simulink model "curiosity_i2c_pitch_roll_yaw"  (R2025b)
settings: Solver=FixedStepDiscrete  StartTime=0.0  StopTime=inf  FixedStep=1e-3  RelTol=1e-3  EnableMultiTasking=on
undefined symbols (not defined in the file): A0, ADC, D10, D7, D8, D9, DiscIntNeverNeededParam, Max, MaxPer, ms, NumBits1, NumBits2, P1, P58, P59, Pin, Resol, s, Timer, us
libraries: MCHP_Blockset x18, simulink x17
(part 1 of 4)
settings Model: SimulationMode=external  ExtModeEnableFloating=off  ExtModeTrigDuration=20  Creator=I52209  LastModifiedBy=I67977
settings SolverCC: AlgebraicLoopSolver=TrustRegion
settings OptimizationCC: DefaultParameterBehavior=Inlined  DefaultUnderspecifiedDataType=single  EnhancedBackFolding=on  BooleansAsBitfields=on  PassReuseOutputArgsAs=Individual arguments  ZeroExternalMemoryAtStartup=off  ZeroInternalMemoryAtStartup=off  OptimizeBlockOrder=speed  DifferentSizesBufferReuse=on  EfficientTunableParamExpr=on
settings DebuggingCC: MultiTaskDSMMsg=none  MultiTaskCondExecSysMsg=none  MultiTaskRateTransMsg=warning  ParameterTunabilityLossMsg=error  ArithmeticOperatorsInVariantConditions=warning
settings HardwareCC: ProdBitPerPointer=32.0  ProdBitPerSizeT=32.0  ProdBitPerPtrDiffT=32.0  ProdLargestAtomicInteger=Long  ProdWordSize=32.0  ProdLongLongMode=on  ProdHWDeviceType=Generic->Custom
settings ModelReferenceCC: ModelReferenceNumInstancesAllowed=Single
settings SFSimCC: MATLABDynamicMemAlloc=off  CustomCodeUndefinedFunction=UseInterfaceOnly
settings RTWCC: SystemTargetFile=MCHP_dsPIC33A_noTMF_stf.tlc  TLCOptions="-aExtModeXCPClassicInterface=0  -aCreateExtModeTypes=1 -aExtModeXCPSimulationTimeInTicks=1"  TemplateMakefile=MCHP_dsPIC33A.tmf  Toolchain=MPLAB XC-DSC - v3.21 for dsPIC DSCs (Microchip)  BuildConfiguration=Specify  GPUComputeCapability=3.5  Description=Microchip Embedded Target dsPIC33A no TMF (real-time)
settings CodeAppCC: ForceParamTrailComments=on  IgnoreCustomStorageClasses=off  MaxIdLength=255.0  OperatorAnnotations=on  SimulinkDataObjDesc=on  SFDataObjDesc=on  InsertBlockDesc=on
settings STFCustomTargetCC: SystemTargetFile=MCHP_dsPIC33A_noTMF_stf.tlc  TargetLangStandard=C99 (ISO)  MultiwordLength=256.0  ConcurrentExecutionCompliant=off  CombineOutputUpdateFcns=on  CombineSignalStateStructs=on  ERTCustomFileBanners=on  SupportContinuousTime=off  RemoveResetFunc=on  MATLABClassNameForMDSCustomization=Simulink.SoftwareTarget.ERTCustomization  GRTInterface=off  UseToolchainInfoCompliant=on  TIMER_PERIOD="[0  49999  65535]"  LDFLAGS='--report-mem,-Map=$(PRODUCT_NAME).map,-cref,-lq-dsp,--memorysummary,memoryfile.xml'  TIMER_START="[0  3  0]"  MCHP_MULTITHREAD_COMPILATION=on  OPTIM_GCC=-O2 -fno-short-double -mno-eds-warn -mconst-in-data -mlarge-code -mlarge-data -mlarge-aggregate -g -Wa,--reorder  OBJDUMP=xc-dsc-objdump  RTWGenSettings_txt="s.UART_TX_IMPLEMENTATION='[2]';s.UART_RX_IMPLEMENTATION='[2]';s.UART_TX_DMACHANNEL='[0]';s.UART_HALF_DUPLEX_MODE='[0]';s.UART_TX_THREAD_PROTECTION='[9]';s.RefMasterBlk='curiosity_i2c_pitch_roll_yaw/CuriosityPlatform Development Board dsPIC33AK128MC106 GP DIM/Microchip Master';s.ChipIdN='[33  128  106]';s.ChipIdL1='AK';s.ChipIdL2='MC';s.ChipIdL3=' ';s.arch3='33A';s.ChipId='33AK128MC106';s.Arch='8';s.bitFieldsSFR='3';s.ChipRAM='16384';s.ChipRAM_XBegin='16384';s.ChipRAM_dma='[-1 -1]';s.FuseConfigTxt='#pragma config FWDT_WDTEN = SW\\\\n#pragma config FICD_JTAGEN = OFF\\\\n#pragma config FDEVOPT_ALTI2C2 = ON\\\\n';s.TimeStep_Timer='2';s.TimeStep_SyncADC='1';s.ADPCFG='0';s.ANSEL_Exist='1';s.ANSEL='[4031   975    -1    -1    -1    -1    -1    -1    -1    -1    -1]';s.TRIS='[65535  65535  63495  65535     -1     -1     -1     -1     -1     -1     -1     -1     -1     -1     -1     -1     -1     -1     -1     -1     -1     -1     -1     -1     -1     -1     -1     -1     -1     -1     -1     -1     -1     -1     -1     -1     -1     -1     -1     -1     -1     -1     -1     -1     -1     -1     -1     -1     -1     -1     -1     -1     -1     -1     -1     -1     -1]';s.RPOR='[-1    -1    -1    -1    -1    -1    -1    -1    -1    -1    -1    -1    -1    -1  2304    -1    -1    -1    -1    -1]';s.RPINR='[-1  -1  -1  -1  -1  -1  -1  -1  -1  59  -1  -1  -1  -1  -1  -1  -1  -1  -1  -1  -1  -1]';s.LATSET='[-1 -1 -1 -1 -1 -1 -1 -1 -1 -1 -1 -1 -1 -1 -1 -1 -1 -1 -1 -1 -1 -1 -1 -1 -1 -1 -1 -1 -1 -1 -1 -1 -1 -1 -1 -1 -1 -1 -1 -1 -1 -1 -1 -1 -1 -1 -1 -1 -1 -1 -1 -1 -1 -1 -1 -1 -1]';s.LATCLR='[-1 -1 -1 -1 -1 -1 -1 -1 -1 -1 -1 -1 -1 -1 -1 -1 -1 -1 -1 -1 -1 -1 -1 -1 -1 -1 -1 -1 -1 -1 -1 -1 -1 -1 -1 -1 -1 -1 -1 -1 -1 -1 -1 -1 -1 -1 -1 -1 -1 -1 -1 -1 -1 -1 -1 -1 -1]';s.ODC='[-1 -1 -1 -1 -1 -1 -1 -1 -1 -1 -1 -1 -1 -1 -1 -1 -1 -1 -1 -1 -1 -1 -1 -1 -1 -1 -1 -1 -1 -1 -1 -1 -1 -1 -1 -1 -1 -1 -1 -1 -1 -1 -1 -1 -1 -1 -1 -1 -1 -1 -1 -1 -1 -1 -1 -1 -1]';s.CNPU='[-1 -1 -1 -1 -1 -1 -1 -1 -1 -1 -1 -1 -1 -1 -1 -1 -1 -1 -1 -1 -1 -1 -1 -1 -1 -1 -1 -1 -1 -1 -1 -1 -1 -1 -1 -1 -1 -1 -1 -1 -1 -1 -1 -1 -1 -1 -1 -1 -1 -1 -1 -1 -1 -1 -1 -1 -1]';s.CNPD='[-1 -1 -1 -1 -1 -1 -1 -1 -1 -1 -1 -1 -1 -1 -1 -1 -1 -1 -1 -1 -1 -1 -1 -1 -1 -1 -1 -1 -1 -1 -1 -1 -1 -1 -1 -1 -1 -1 -1 -1 -1 -1 -1 -1 -1 -1 -1 -1 -1 -1 -1 -1 -1 -1 -1 -1 -1]';s.PortConfigTxt=' ';s.CLKDIV='0';s.PLLFBD='-1';s.PLLDIV='16815713';s.QUARTZ='8000000';s.SWITCH_OSC='16386';s.PLLRNG='-1';s.MASTER_BusyFlag='-1';s.POWERSAVE='0';s.MIPS='200000000';s.FLASH_ECC='0';s.PBxDIV='[-1]';s.CLKx_INTDIV='[-1 -1 -1 -1  0  1 -1  0  0 -1 -1  0 -1]';s.CLKx_FRACDIV='[-1   -1   -1   -1    0  256   -1    0    0   -1   -1    0   -1]';s.AN_type2='1';s.ACLKCON_reg='-1';s.nTIMERS='1';s.nSCCP='4';s.DOS_04094_cpu_33a_v1_dspic33a='1';s.DOS_04436_perseus_dspic33a='1';s.DOS_04928_gpio_ports_upb_v2_dspic33a='1';s.DOS_02672_math_progcrc_upb_v1_dspic33a='1';s.DOS_04993_sec_32bit_cp_upb_v1_dspic33a='1';s.DOS_03459_adc_pc_ctrl_upb_v2_dspic33a='1';s.DOS_04302_pwm_pc_upb_v3_dspic33a='1';s.DOS_03076_uart_protocol_upb_v1_dspic33a='1';s.DOS_01482_spi_i2s_upb_v1_dspic33a='1';s.DOS_05155_i2c_upb_v4_dspic33a='1';s.DOS_02359_sent_j2716_upb_v1_dspic33a='1';s.DOS_05177_qei_32b_upb_v2_dspic33a='1';s.DOS_01512_ccp_mccp_upb_v1_dspic33a='1';s.DOS_03496_dac_pdm_nbit_upb_v2_dspic33a='1';s.DOS_02673_tmr_classa_upb_v1_dspic33a='1';s.DOS_04776_perf_mon_upb_v1_dspic33a='1';s.DOS_03680_pfm_pbu_33a_upb_v1_dspic33a='1';s.DOS_04649_sec_pac_upb_v0_dspic33a='1';s.DOS_03966_io_integrity_monitor_upb_v1_dspic33a='1';s.DOS_04641_biss_master_upb_v1_dspic33a='1';s.DOS_04077_dma_upb_v1_dspic33a='1';s.DOS_04549_nvm_ctrl_32bit_upb_v1_dspic33a='1';s.DOS_04449_clk_cru_33a_upb_v1_dspic33a='1';s.DOS_03850_clk_monitor_upb_v1_dspic33a='1';s.DOS_04342_osc_rc8mhz_ctrl_upb_v4_dspic33a='1';s.DOS_04650_wdt_upb_v4_dspic33a='1';s.DOS_05178_ptg_pc_upb_v2_dspic33a='1';s.DOS_04181_data_ram_ctrl_upb_v1_dspic33a='1';s.DOS_04735_wdt_dmt_upb_v6_dspic33a='1';s.DOS_01577_cla_clc_upb_v1_dspic33a='1';s.DOS_03516_pwr_sib_upb_v3_dspic33a='1';s.DOS_03495_amp_pad_opamp_ctrl_upb_v2_dspic33a='1';s.DOS_05308_pegasus_dspic33a='0';s.DOS_02976_adc_12b_upb_v2_dspic33a='0';s.DOS_05404_adc_pc_ctrl_upb_v3_dspic33a='0';s.DOS_05226_pwm_pc_upb_v4_dspic33a='0';s.DOS_05226_apwm_pc_upb_v4_dspic33a='0';s.DOS_05431_dac_pdm_nbit_upb_v3_dspic33a='0';s.DOS_04649_sec_pac_upb_v1_dspic33a='0';s.DOS_05461_pwr_sib_upb_v4_dspic33a='0';s.DOS_05420_amp_vref_ctl_upb_v1_dspic33a='0';s.DOS_05346_sec_cam_v2_dspic33a='0';s.DOS_03267_adc_soft_code_seq_v1_dspic33a='0';s.DOS_04537_can_fd_upb_v3_dspic33a='0';s.DOS_05557_serpens_dspic33a='0';s.DOS_05972_adc_12b_upb_v3_adc_dspic33a='0';s.DOS_03681_bmx_33a_upb_v1_dspic33a='0';s.DOS_05514_qei_32b_upb_v3_dspic33a='0';s.DOS_02050_tmr_rtcc_upb_v1_dspic33a='0';s.DOS_04649_sec_pac_upb_serpens_dspic33a='0';s.DOS_05801_dma_upb_v2_dspic33a='0';s.DOS_05692_pwr_sib_upb_v5_dspic33a='0';s.DOS_06006_adc_soft_code_seq_v2_adc_dspic33a='0';s.DOS_05442_icd_trace_33a_v1_dspic33a='0';s.DOS_02551_cpu_16bit_v7='0';s.DOS_01520_wdt_dmt_upb_v1_16bit='0';s.DOS_02359a_sent_j2716_upb_v1='0';s.DOS_02672_math_progcrc_upb_v1_16bit='0';s.DOS_01577_cla_clc_upb_v1='0';s.DOS_02915_ecc_v2='0';s.DOS_02673_tmr_classa_upb_v1_16bit='0';s.DOS_01494_qei_32b_upb_v1_16bit='0';s.DOS_02472_ppi_pmp16_upb_v1_16bit='0';s.DOS_01441_i2c_upb_v1_16bit_TLAH='0';s.DOS_03076_uart_protocol_upb_v1_16bit='0';s.DOS_01482='0';s.DOS_01483_pwm_16bit='0';s.DOS_02949_WACG='0';s.DOS_02316_nvm_ctrl_v1_16bit='0';s.DOS_03349_amp_pad_opamp_ctrl_upb_v1='0';s.DOS_02653_afe_current_bias_ctrl_upb_v1_16bit='0';s.DOS_01459_ptg_pc_upb_v1_16bit='0';s.DOS_01512_ccp_mccp_upb_v1_16bit='0';s.DOS_02519_dma_sfr_16bit_v2='0';s.DOS_02508c11='0';s.DOS_02475_dac_pdm_nbit_upb_v1_16bit='0';s.DOS_02467_gpio_upb_v1_16bit='0';s.DOS_00805_rst_integration_v4='0';s.DOS_02659_clk_sib_v12='0';s.DOS_02237_osc_dco_ctrl_upb_v1_16bit='0';s.DOS_02674_wdt_upb_v1_16bit='0';s.DOS_01407='0';s.DOS_03247_CAN_FD_UPB_V2_16_bit='0';s.DOS_03994_WAC07='0';s.DOS_02552_msi_upb_v1_Master='0';s.DOS_03667_pwm_pc_upb_v2_16bit='0';s.DOS_04180_drm_ctrl_ecc_v1='0';s.DOS_03431_STX03='0';s.DOS_03516_pwr_sib_upb_v3='0';s.DOS_02552_msi_upb_v1_Slave='0';s.DOS_04621_amp_pga_ctrl_upb_v3='0';s.DOS_02497_WACV='0';s.DOS_02593_amp_pga_ctrl_pb_v2_16bit='0';s.DOS_01461_afe_ctmu_con_upb_v1_16bit='0';s.DOS_02497_WACA='0';s.DOS_02478_uart_irda_upb_v1_16bit='0';s.DOS_00929='0';s.DOS_01198='0';s.DOS_03029_WACH='0';s.DOS_01483_apwm_16bit='0';s.DOS_04797_WAC0A='0';s.DOS_04884_WAC0B='0';s.DOS_04797_WAC09='0';s.DOS_03662_WACU='0';s.DOS_00794='0';s.DOS_00931='0';s.DOS_00932='0';s.DOS_00942='0';s.DOS_00938='0';s.DOS_00996='0';s.DOS_00997='0';s.DOS_00998='0';s.DOS_00209='0';s.DOS_01555_adc='0';s.DOS_01293='0';s.DOS_00828='0';s.DOS_01116='0';s.DOS_01017_RPORx='0';s.DOS_01017_RPINRx='0';s.DOS_01555_nvm_tsmc18_v2_16bit='0';s.DOS_00804='0';s.DOS_00826='0';s.DOS_01555_TLAK_PMDx='0';s.DOS_01555_TLAK_INT_='0';s.DOS_00933='0';s.DOS_01555='0';s.DOS_01555_ptg='0';s.DOS_00958='0';s.DOS_01117_PORTx='0';s.DOS_00999='0';s.DOS_01041='0';s.DOS_00892='0';s.DOS_01287_TLAC_PMDx='0';s.DOS_01287_TLAC_INT_='0';s.DOS_01424='0';s.DOS_01332='0';s.DOS_01468_PMBA_current_source='0';s.DOS_02291_PGA='0';s.DOS_01467_Comparator='0';s.DOS_01498_TLAY='0';s.DOS_00993_PLL_120MHz='0';s.DOS_01332_ptg_pc_v1='0';s.DOS_00958_pwm_TLAY='0';s.TLAY_IOPorts='0';s.DOS_00929q='0';s.DOS_02415_spi_v5='0';s.DOS_RPINRx_16bit_2='0';s.DOS_01497_TLAH_PMDx='0';s.DOS_02550_TLAL_INT='0';s.DOS_00958_pwm_TLAH='0';s.DOS_01287_TLAH_INT_='0';s.DOS_01113='0';s.DOS_01017_PMDx='0';s.DOS_00927='0';s.DOS_01080='0';s.DOS_00794_cpu_16bit_v3='0';s.DOS_02192_TLCD_PMDx='0';s.DOS_02192_TLCD_INT_='0';s.DOS_02192_cmp='0';s.DOS_00958_pwm_TLCD='0';s.DOS_02192_PORTx_TLCD='0';s.DOS_00936='0';s.DOS_00995='0';s.DOS_00546='0';s.DOS_00474='0';s.DOS_02481_WACP_Config='0';s.DOS_03088_pfm_cache_ocp_v2_WACK='0';s.DOS_02819_pfm_ctrl_32bit_upb_v2='0';s.DOS_02674_wdt_upb_v1_32bit='0';s.DOS_01520_wdt_dmt_upb_v1='0';s.DOS_02869_icd_jtag_bvci_upb_v2='0';s.DOS_02823_WACJ_clk_cru_upb_v2='0';s.DOS_02823_WACN_clk_cru_upb_v2='0';s.DOS_01423_RPINRx='0';s.DOS_02481_RPORx='0';s.DOS_02511_pwr_sib_upb_v1_32bit='0';s.DOS_02907_WACP_int_evic_v3='0';s.DOS_01500_dma_bvci_v2='0';s.DOS_02141_tmr_classa_pb_v2='0';s.DOS_02815_tmr_classb_upb_v1='0';s.DOS_00740_icap_pb_v1='0';s.DOS_00749_ocmp_pb_v1='0';s.DOS_01441_i2c_upb_v1_32bit='0';s.DOS_01329_spi_pb_v2='0';s.DOS_02478_uart_irda_upb_v1_32bit='0';s.DOS_01477_pwm_mc_upb_v1='0';s.DOS_01494_qei_32b_upb_v1='0';s.DOS_03554_cmp_control_upb_v2_32bit='0';s.DOS_01445_dac_nbit__control_upb_v1_32bit='0';s.DOS_01461_afe_ctmu_con_upb_v1='0';s.DOS_01577_cla_clc_upb_v1_32bit='0';s.DOS_02467_gpio_ports_upb_v1='0';s.DOS_02508_WACP_adc_sar_ctrl_upb_v1='0';s.DOS_01261_tmr_rtcc_WACJ_K_N_P_pb_v2='0';s.DOS_EIP_00136_ssx_v1='0';s.DOS_02481_WACK_MC_Config='0';s.DOS_02907_WACN_GP_int_evic_v3='0';s.DOS_02508_adc_sar_ctrl_upb_v1_PIC32MK='0';s.DOS_01261_tmr_rtcc_pb_v2='0';s.DOS_01475_lpwr_deep_sleep_ctrl_v2='0';s.DOS_02907_WACN_MC_int_evic_v3='0';s.DOS_03247_can_fd_upb_v2_pic32mk='0';s.DOS_02907_WACK_MC_int_evic_v3='0';s.DOS_02514_dfm_strl_sst_upb_v1='0';s.DOS_02472_ppi_pmp16_upb_v1='0';s.DOS_02813a_usb_otgcore_pb_v3='0';s.DOS_02481_WACJ_MC_Config='0';s.DOS_02569_pfm_cache_ocp_v1='0';s.DOS_02481_WACJ_MC_int_evic_v3='0';s.DOS_01459_ptg_pc_upb_v1_SIC='0';s.DOS_01427_cmp_control_upb_v1_32bit='0';s.DOS_01152_can_bvci_v1='0';s.DOS_02787_WACD_Config='0';s.DOS_00800_dac_4bit_ctrl_pb_v1='0';s.DOS_01539_icd_jtag_pb_v2='0';s.DOS_02823_clk_cru_upb_v2='0';s.DOS_01423_RPORx='0';s.DOS_02907_WACD_int_evic_v3='0';s.DOS_00734_uart_irda_pb_v1='0';s.DOS_00687_tmr_classa_pb_v1='0';s.DOS_00745_tmr_classb_pb_v1='0';s.DOS_02508_adc_sar_ctrl_upb_v1='0';s.DOS_00866_cmp_control_pb_v2='0';s.DOS_01114_eth_bvci_v1='0';s.DOS_02831_usb_clk_rst_v2='0';s.DOS_01643_pfm_cache_ahb_v2='0';s.DOS_EIP_00206r5_sqi_v2='0';s.DOS_EIP_00124_usb_hs_otgcore_v1='0';s.DOS_EIP_00218_math_rng_ahbs_v2='0';s.DOS_EIP_00109_ebi_v1='0';s.DOS_EIP_00158_crypto_v1='0';"  PIC_REF=33AK128MC106  BIN2HEX=xc-dsc-bin2hex  AR1=xc-dsc-ar  GCCPATH=C:/PROGRA~1/MICROC~1/xc-dsc/v3.21/bin  MCHP_AUTO_FLASH=off  LINKER_SCRIPT=p33AK128MC106.gld  MCHP_XCP_MemoryBlockParameters=[-1 8]  AssemblyListing=on  LinkWithMaster=off  TIMER_PRESCALER="[-1  1  1 -1 -1]"  ProduceHexOutput=off  EXTMODE_DATA_UPLOAD=on  HOST_PLATFORM=PC  GCC1=xc-dsc-gcc.exe
settings ERTTargetCC: ExtMode=on  ExtModeTransport=1.0  ExtModeStaticAlloc=on  ExtModeMaxTrigDuration=20.0  ExtModeStaticAllocSize=2048.0  ExtModeMexFile=ext_xcp  ExtModeMexArgs=1 21 460800 './curiosity_i2c_pitch_roll_yaw.X/curiosity_i2c_pitch_roll_yaw.elf'  ExtModeIntrfLevel=Level2 - Open  ERTSrcFileBannerTemplate=MCHP_dsPIC_code_template.cgt  ERTHdrFileBannerTemplate=MCHP_dsPIC_code_template.cgt  ERTDataSrcFileTemplate=MCHP_dsPIC_code_template.cgt  ERTDataHdrFileTemplate=MCHP_dsPIC_code_template.cgt  ERTCustomFileTemplate=MCHP_main.tlc  MaxLineWidth=110.0  TargetLangStandard=C99 (ISO)  ParMdlRefBuildCompliant=off  CompOptLevelCompliant=off  ConcurrentExecutionCompliant=off  CombineSignalStateStructs=on  SupportNonInlinedSFcns=on  ModelStepFunctionPrototypeControlCompliant=off  CPPClassGenCompliant=off

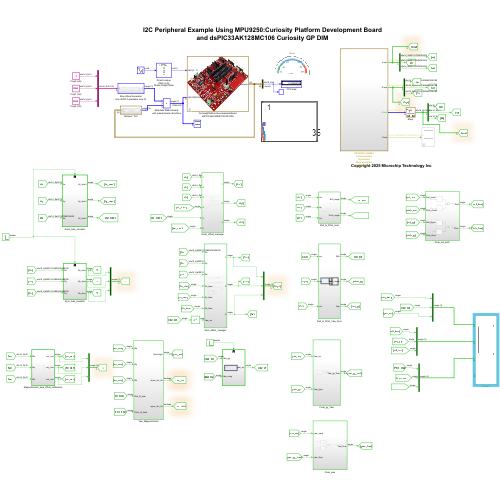
[thumbnail: Simulink's stored preview of the top-level diagram]
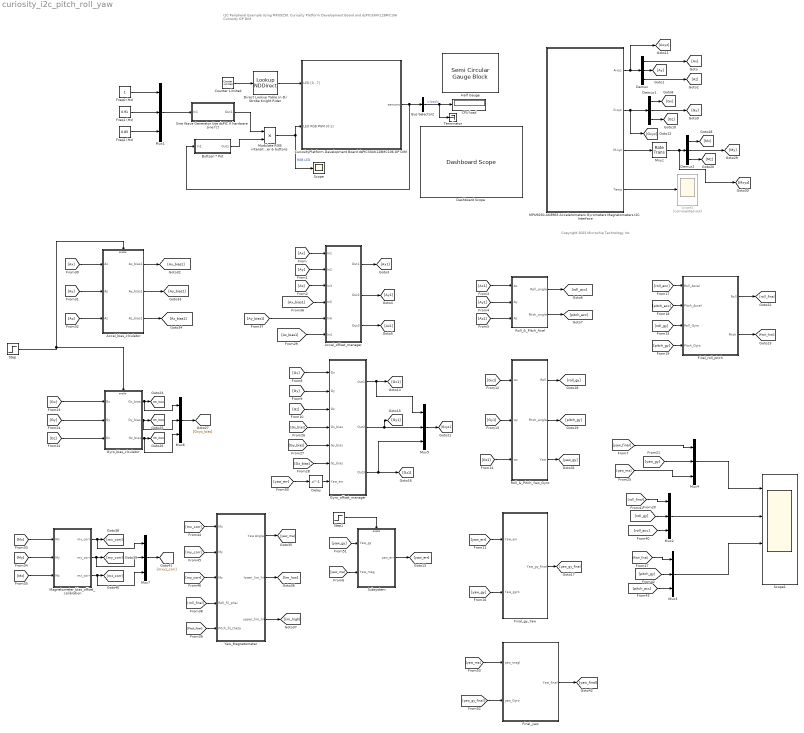
== system curiosity_i2c_pitch_roll_yaw ==
  note: Copyright 2025 Microchip Technology Inc
  note: I2C Peripheral Example Using MPU9250: Curiosity Platform Development Board and dsPIC33AK128MC106 Curiosity GP DIM
  Accel_bias_clculator : Subsystem  TreatAsAtomicUnit=on
  Accel_offset_manager : Subsystem
  Bus Selector2 : BusSelector  OutputSignals=MCU.load
  Buttosn * Pot : Subsystem
  CPU load : Display
  Counter Limited : simulink/Sources/Counter Limited  uplimit=13  tsamp=0.05
  CuriosityPlatform Development Board dsPIC33AK128MC106 GP DIM : Subsystem
      mask Display: image('MCHP_i_Board_Curiosity_dsPICA.jpg')
  Dashboard Scope : DashboardScope  TimeSpan=5  Ymin=0  Ymax=1  LegendPosition=Hide  ScaleAtStop=off  TicksPosition=Inside  FontColor=[0.0, 0.0, 0.0]
  Delay : Delay  DelayLength=1
  Demux : Demux  Outputs=3
  Demux1 : Demux  Outputs=3
  Demux2 : Demux  Outputs=3
  Direct Lookup Table (n-D) Strobe Knight Rider : LookupNDDirect  NumberOfTableDimensions=1  Table=uint16(2.^[[0:7] [6:-1:1]] )  RemoveProtectionInput=on
  Final_gy_Yaw : Subsystem
  Final_roll_pitch : Subsystem
  Final_yaw : Subsystem
  Freq0 (Hz) : Constant  OutDataTypeStr=fixdt(0,16,10)
  Freq1 (Hz) : Constant  Value=0.91  OutDataTypeStr=fixdt(0,16,10)
  Freq2 (Hz) : Constant  Value=0.85  OutDataTypeStr=fixdt(0,16,10)
  Gyro_bias_clculator : Subsystem  TreatAsAtomicUnit=on
  Gyro_offset_manager : Subsystem
  Half Gauge : SemiCircularGaugeBlock  FontColor=[0.0, 0.0, 0.0]
  MPU9250-AK8963 Accelerometers Gyrometers Magnetometers I2C Interface : Subsystem
  Magnetometer_bias_offset_calibration : Subsystem  TreatAsAtomicUnit=on
  Modulate RGB intensity with potentiometer & buttons : Product  OutDataTypeStr=single
  Mux{1..7} (7 alike) : Mux  Inputs=3
  Mxyz : RateTransition  Deterministic=off  OutPortSampleTimeOpt=Inherit
  Roll_&_Pitch_Acel : Subsystem
  Roll_&_Pitch_Yaw_Gyro : Subsystem
  Scope : Scope
      settings: ActiveDisplayYMinimum=-0.06269  ActiveDisplayYMaximum=0.5642
  Scope1 : Scope  NumInputPorts=4
      settings: ActiveDisplayYMinimum=-0.37342479638755322  ActiveDisplayYMaximum=0.911760849878192  DataLoggingVariableName=ScopeData2
  Scope2 : Scope  Commented=on
      settings: ActiveDisplayYMinimum=19.60574  ActiveDisplayYMaximum=33.5483  DataLoggingVariableName=ScopeData3
  Sine Wave Generator Use dsPIC A hardware sine fct : Subsystem
  Step : Step  Time=2  Before=1  After=0  SampleTime=0.005
  Step1 : Step  Time=2  Before=1  After=0  SampleTime=0.005
  Subsystem : Subsystem
  Terminator : Terminator
  Yaw_Magnetometer : Subsystem
  wires:
  [Gy] -> Gyro_offset_manager/2(Gy)
  [yaw_gy] -> Mux4/2
  [Ay] -> Accel_offset_manager/2(In2)
  [Gz] -> Gyro_offset_manager/3(Gz)
  MPU9250-AK8963 Accelerometers Gyrometers Magnetometers I2C Interface/2(G-xyz) -> [Gxyz], Demux1/1
  [Gy] -> Gyro_bias_clculator/2(Gy)
  Yaw_Magnetometer/3(upper_lim_hit) -> [lim_high]
  [Az1] -> Roll_&_Pitch_Acel/3(Az)
  Demux1/2 -> [Gy]
  Mux6/1 -> [Gxyz_bias]
  [yaw_ma] -> Final_yaw/1(yaw_magl)
  [yaw_gy] -> Subsystem/1(Yaw_gy)
  [pitch_gy] -> Final_roll_pitch/4(Pitch_Gyro)
  Magnetometer_bias_offset_calibration/3(mz_corr) -> Mux7/3, [mz_corr]
  [roll_final] -> Mux2/1
  Counter Limited/1 -> Direct Lookup Table (n-D) Strobe Knight Rider/1
  [Ay_bias1] -> Accel_offset_manager/5(In6)
  [yaw_ma] -> Mux4/3
  [Gz] -> Gyro_bias_clculator/3(Gz)
  [Gx_bias] -> Gyro_offset_manager/4(Gx_bias)
  [mz_corr] -> Yaw_Magnetometer/3(Mz)
  Yaw_Magnetometer/1(Yaw Angle) -> [yaw_ma]
  Accel_bias_clculator/2(Ay_bias1) -> [Ay_bias1]
  Demux2/1 -> [Mx]
  [mx_corr] -> Yaw_Magnetometer/1(Mx)
  [yaw_gy_final] -> Final_yaw/2(yaw_Gyro)
  Demux2/2 -> [My]
  [yaw_ma] -> Subsystem/2(Yaw_mag)
  Sine Wave Generator Use dsPIC A hardware sine fct/1(Out1) -> Modulate RGB intensity with potentiometer & buttons/1
  Final_yaw/1(Yaw_final) -> [yaw_final]
  Demux1/1 -> [Gx]
  Gyro_bias_clculator/1(Gx_bias) -> Mux6/1, [Gx_bias]
  [roll_gy] -> Mux2/2
  [Ax] -> Accel_offset_manager/1(In1)
  Buttosn * Pot/1(Out1) -> Modulate RGB intensity with potentiometer & buttons/2
  Modulate RGB intensity with potentiometer & buttons/1 -> CuriosityPlatform Development Board dsPIC33AK128MC106 GP DIM/2(LED RGB PWM [0-1]), Scope/1  "RGB LED"
  Roll_&_Pitch_Yaw_Gyro/3(Yaw) -> [yaw_gy]
  [roll_acc] -> Mux2/3
  Freq2 (Hz)/1 -> Mux1/3
  Final_gy_Yaw/1(Yaw_gy_final) -> [yaw_gy_final]
  Freq0 (Hz)/1 -> Mux1/1
  Step/1 -> Accel_bias_clculator/Enable, Gyro_bias_clculator/Enable
  [Az] -> Accel_offset_manager/3(In3)
  [pitch_acc] -> Final_roll_pitch/2(Pitch_Accel)
  Magnetometer_bias_offset_calibration/2(my_corr) -> Mux7/2, [my_corr]
  [Gz_bias] -> Gyro_offset_manager/6(Gz_bias)
  [pitch_acc] -> Mux3/3
  Yaw_Magnetometer/2(lower_lim_hit) -> [lim_low]
  Demux2/3 -> [Mz]
  Gyro_offset_manager/2(Out2) -> [Gy1], Mux5/2
  [My] -> Magnetometer_bias_offset_calibration/2(My)
  Step1/1 -> Subsystem/Enable
  Demux/2 -> [Ay]
  Gyro_offset_manager/1(Out1) -> [Gx1], Mux5/1
  [yaw_err] -> Final_gy_Yaw/1(Yaw_err)
  Mxyz/1 -> [Mxyz], Demux2/1
  CuriosityPlatform Development Board dsPIC33AK128MC106 GP DIM/1(sensors) -> Buttosn * Pot/1(In1), Bus Selector2/1
  [Gy_bias] -> Gyro_offset_manager/5(Gy_bias)
  [roll_gy] -> Final_roll_pitch/3(Roll_Gyro)
  Accel_bias_clculator/1(Ax_bias1) -> [Ax_bias1]
  [Mz] -> Magnetometer_bias_offset_calibration/3(Mz)
  [Az] -> Accel_bias_clculator/3(Az)
  Roll_&_Pitch_Acel/1(Roll_angle) -> [roll_acc]
  [Az_bias1] -> Accel_offset_manager/6(In4)
  Mux4/1 -> Scope1/1
  [roll_final] -> Yaw_Magnetometer/4(Roll_fil_phai)
  Bus Selector2/1 -> Terminator/1, CPU load/1  "<load>"
  [my_corr] -> Yaw_Magnetometer/2(My)
  [yaw_final] -> Mux4/1
  [Gy1] -> Roll_&_Pitch_Yaw_Gyro/2(wy)
  Demux1/3 -> [Gz]
  [Gx] -> Gyro_bias_clculator/1(Gx)
  [Ax_bias1] -> Accel_offset_manager/4(In5)
  Roll_&_Pitch_Yaw_Gyro/2(Pitch_angle) -> [pitch_gy]
  Gyro_bias_clculator/3(Gz_bias) -> Mux6/3, [Gz_bias]
  Mux3/1 -> Scope1/3
  [Pitch_final] -> Yaw_Magnetometer/5(Pitch_fil_theta)
  Magnetometer_bias_offset_calibration/1(mx_corr) -> Mux7/1, [mx_corr]
  Accel_offset_manager/1(Out1) -> [Ax1]
  [Ax1] -> Roll_&_Pitch_Acel/1(Ax)
  [Mx] -> Magnetometer_bias_offset_calibration/1(Mx)
  Accel_offset_manager/3(Out3) -> [Az1]
  [Ax] -> Accel_bias_clculator/1(Ax)
  [yaw_err] -> Delay/1
  Demux/3 -> [Az]
  Subsystem/1(yaw_err) -> [yaw_err]
  Mux1/1 -> Sine Wave Generator Use dsPIC A hardware sine fct/1(In1)
  [Gx] -> Gyro_offset_manager/1(Gx)
  Roll_&_Pitch_Yaw_Gyro/1(Roll) -> [roll_gy]
  MPU9250-AK8963 Accelerometers Gyrometers Magnetometers I2C Interface/3(M-xyz) -> Mxyz/1
  Gyro_bias_clculator/2(Gy_bias) -> Mux6/2, [Gy_bias]
  Mux2/1 -> Scope1/2
  MPU9250-AK8963 Accelerometers Gyrometers Magnetometers I2C Interface/1(A-xyz) -> Demux/1, [Axyz]
  [yaw_gy] -> Final_gy_Yaw/2(Yaw_gyro)
  [Ay] -> Accel_bias_clculator/2(Ay)
  [Gz1] -> Roll_&_Pitch_Yaw_Gyro/3(wz)
  Demux/1 -> [Ax]
  [Gx1] -> Roll_&_Pitch_Yaw_Gyro/1(wx)
  [Pitch_final] -> Mux3/1
  MPU9250-AK8963 Accelerometers Gyrometers Magnetometers I2C Interface/4(Temp) -> Scope2/1
  Direct Lookup Table (n-D) Strobe Knight Rider/1 -> CuriosityPlatform Development Board dsPIC33AK128MC106 GP DIM/1(LED [0...7])
  Delay/1 -> Gyro_offset_manager/7(Yaw_err)
  Final_roll_pitch/2(Pitch) -> [Pitch_final]
  Accel_bias_clculator/3(Az_bias1) -> [Az_bias1]
  Final_roll_pitch/1(Roll) -> [roll_final]
  Freq1 (Hz)/1 -> Mux1/2
  Accel_offset_manager/2(Out2) -> [Ay1]
  [pitch_gy] -> Mux3/2
  Roll_&_Pitch_Acel/2(Pitch_angle) -> [pitch_acc]
  Gyro_offset_manager/3(Out3) -> Mux5/3, [Gz1]
  Mux5/1 -> [Gxyz1]
  [roll_acc] -> Final_roll_pitch/1(Roll_Accel)
  Mux7/1 -> [mxyz_corr]
  [Ay1] -> Roll_&_Pitch_Acel/2(Ay)

== system curiosity_i2c_pitch_roll_yaw/Accel_bias_clculator ==
  Ax : Inport
  Ay : Inport  Port=2
  Az : Inport  Port=3
  Enable : EnablePort
  manu_mean : Subsystem
  manu_mean3 : Subsystem
  manu_mean4 : Subsystem
  Ax_bias1 : Outport
  Ay_bias1 : Outport  Port=2
  Az_bias1 : Outport  Port=3
  wires:
  Ay/1 -> manu_mean3/1(Ay)
  Ax/1 -> manu_mean/1(Ax)
  Az/1 -> manu_mean4/1(Az)
  manu_mean/1(Ax_bias1) -> Ax_bias1/1
  manu_mean3/1(Ay_bias1) -> Ay_bias1/1
  manu_mean4/1(Ax_bias1) -> Az_bias1/1

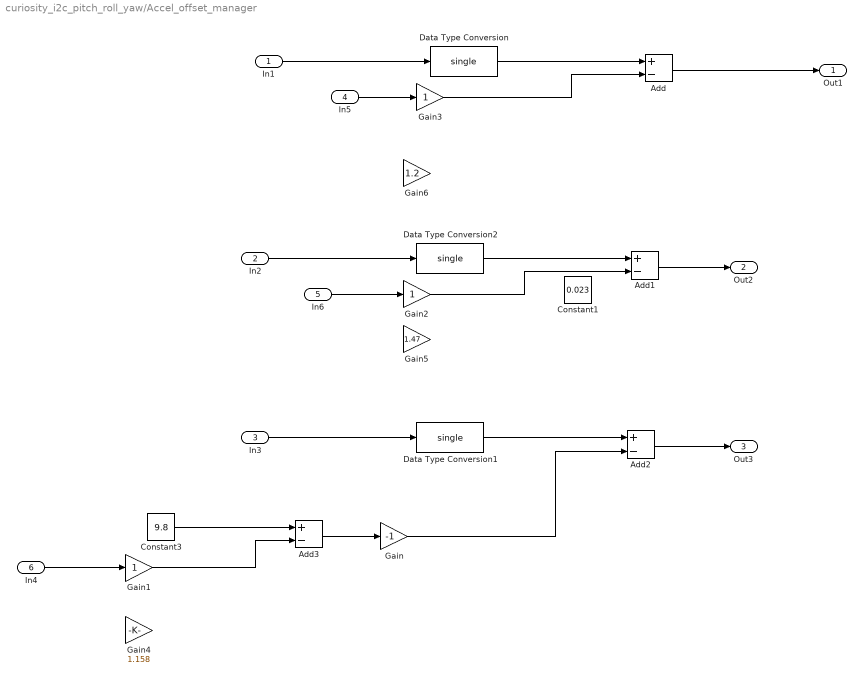
== system curiosity_i2c_pitch_roll_yaw/Accel_offset_manager ==
  In1 : Inport
  In2 : Inport  Port=2
  In3 : Inport  Port=3
  In5 : Inport  Port=4
  In6 : Inport  Port=5
  In4 : Inport  Port=6
  Add : Sum  Inputs=+-  OutDataTypeStr=Inherit: Same as first input
  Add1 : Sum  Inputs=+-  OutDataTypeStr=Inherit: Same as first input
  Add2 : Sum  Inputs=+-  OutDataTypeStr=Inherit: Same as first input
  Add3 : Sum  Inputs=+-
  Constant1 : Constant  Value=0.023  SampleTime=0.005
  Constant3 : Constant  Value=9.8  OutDataTypeStr=single  SampleTime=0.005
  Data Type Conversion : DataTypeConversion  OutDataTypeStr=single  SaturateOnIntegerOverflow=off  RndMeth=Floor
  Data Type Conversion1 : DataTypeConversion  OutDataTypeStr=single  SaturateOnIntegerOverflow=off  RndMeth=Floor
  Data Type Conversion2 : DataTypeConversion  OutDataTypeStr=single  SaturateOnIntegerOverflow=off  RndMeth=Floor
  Gain : Gain  Gain=-1
  Gain1 : Gain
  Gain2 : Gain
  Gain3 : Gain
  Gain4 : Gain  Gain=1.158
  Gain5 : Gain  Gain=1.47
  Gain6 : Gain  Gain=1.2
  Out1 : Outport
  Out2 : Outport  Port=2
  Out3 : Outport  Port=3
  wires:
  In6/1 -> Gain2/1
  Gain2/1 -> Add1/2
  Data Type Conversion2/1 -> Add1/1
  In2/1 -> Data Type Conversion2/1
  Data Type Conversion1/1 -> Add2/1
  In3/1 -> Data Type Conversion1/1
  In1/1 -> Data Type Conversion/1
  Add2/1 -> Out3/1
  Add1/1 -> Out2/1
  Data Type Conversion/1 -> Add/1
  Add/1 -> Out1/1
  Add3/1 -> Gain/1
  Constant3/1 -> Add3/1
  In4/1 -> Gain1/1
  In5/1 -> Gain3/1
  Gain3/1 -> Add/2
  Gain/1 -> Add2/2
  Gain1/1 -> Add3/2

== system curiosity_i2c_pitch_roll_yaw/Buttosn * Pot ==
  In1 : Inport
  Bus Selector : BusSelector  OutputSignals=ADC.pot
  Bus Selector1 : BusSelector  OutputSignals=BTN.S1,BTN.S2,BTN.S3
  Cast1 : DataTypeConversion  OutDataTypeStr=single  SaturateOnIntegerOverflow=off  RndMeth=Floor
  Desactivate R,G or B with buttons 1,2 or 3 multiplied by pot : Product  OutDataTypeStr=single
  Downsample x10 : Subsystem  mask{DownSample=10}
      mask prompts: DownSample "DownSample Factor"
  Mux : Mux  Inputs=3
  Rate Transition : RateTransition
  Out1 : Outport
  wires:
  Mux/1 -> Cast1/1
  Rate Transition/1 -> Desactivate R,G or B with buttons 1,2 or 3 multiplied by pot/2  "U1 CH1"
  In1/1 -> Bus Selector1/1, Bus Selector/1
  Bus Selector1/3 -> Mux/3  "<S3>"
  Downsample x10/1(Out1) -> Rate Transition/1
  Bus Selector/1 -> Downsample x10/1(In1)  "<pot>"
  Desactivate R,G or B with buttons 1,2 or 3 multiplied by pot/1 -> Out1/1
  Bus Selector1/1 -> Mux/1  "<S1>"
  Bus Selector1/2 -> Mux/2  "<S2>"
  Cast1/1 -> Desactivate R,G or B with buttons 1,2 or 3 multiplied by pot/1
